simulink model "Comparison_with_prior_ESC_Methods"  (R2023a)
settings: Solver=ode4  StartTime=0.0  StopTime=500  FixedStep=0.0001  RelTol=1e-6
settings Model: Creator=Ahmed  LastModifiedBy=Ahmed

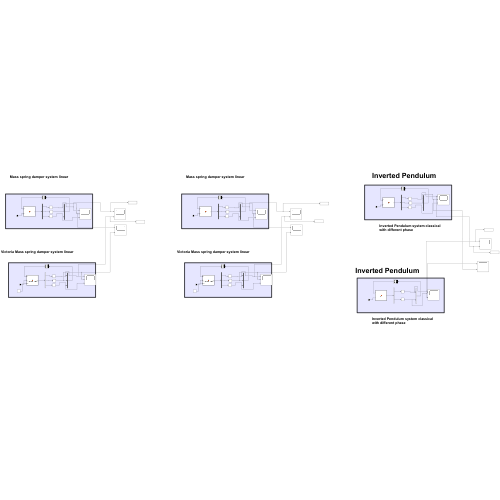
[thumbnail: Simulink's stored preview of the top-level diagram]
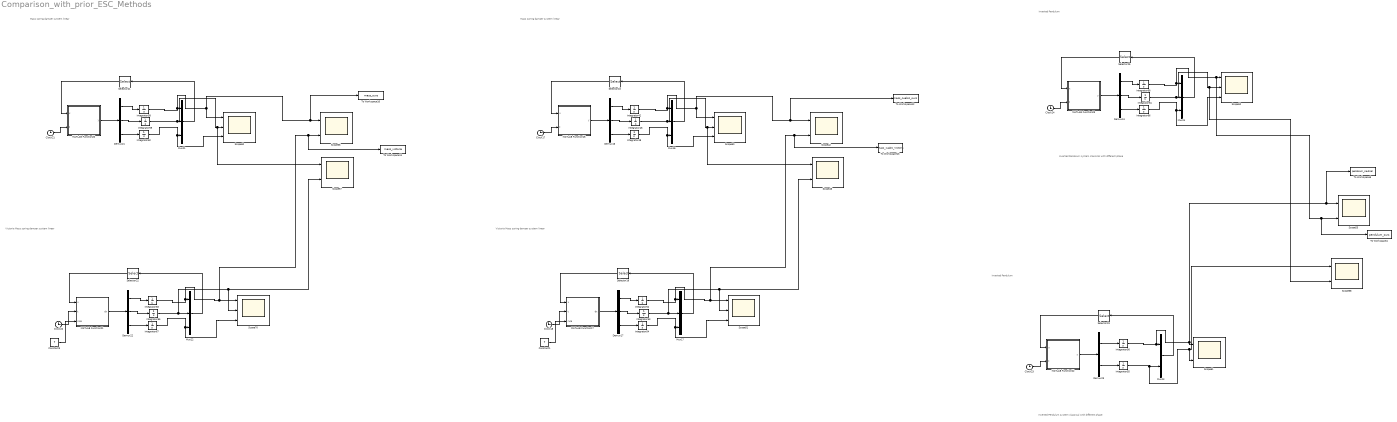
== system Comparison_with_prior_ESC_Methods ==
  note: Mass spring damper system linear
  note: Victoria Mass spring damper system linear
  note: Mass spring damper system linear
  note: Victoria Mass spring damper system linear
  note: Inverted Pendulum system classical with different phase
  note: Inverted Pendulum
  note: Inverted Pendulum system classical with different phase
  note: Inverted Pendulum
  Clock{17..18,21..24} (6 alike) : Clock
  Constant1 : Constant  Value=7
  Constant3 : Constant  Value=7
  Demux{16..17,21..22,24} (5 alike) : Demux  Outputs=3
  Demux23 : Demux  Outputs=2
  Integrator42 : Integrator  InitialCondition=2
  Integrator{46,53,55,59,61,65} (6 alike) : Integrator  InitialCondition=-1
  Integrator{48,54,62,66..67} (5 alike) : Integrator
  Integrator52 : Integrator  InitialCondition=1.68
  Integrator56 : Integrator  InitialCondition=3
  Integrator58 : Integrator  InitialCondition=2
  Integrator63 : Integrator  InitialCondition=1.68
  Integrator68 : Integrator  InitialCondition=3
  MATLAB Function16 : MATLAB Function  TreatAsAtomicUnit=on
  MATLAB Function17 : MATLAB Function  TreatAsAtomicUnit=on
  MATLAB Function20 : MATLAB Function  TreatAsAtomicUnit=on
  MATLAB Function21 : MATLAB Function  TreatAsAtomicUnit=on
  MATLAB Function22 : MATLAB Function  TreatAsAtomicUnit=on
  MATLAB Function23 : MATLAB Function  TreatAsAtomicUnit=on
  Mux{16..17,21..22,24} (5 alike) : Mux  Inputs=3
  Mux23 : Mux  Inputs=2
  Scope{42,46,53,56..58,61} (7 alike) : Scope  NumInputPorts=2
  Scope{50..52,62,70} (5 alike) : Scope  NumInputPorts=3
  Selector{16,19,21..22,25} (5 alike) : Selector  InputPortWidth=3  IndexOptions=Index vector (dialog)  Indices=[1 2 3]  OutputSizes=1
  Selector23 : Selector  InputPortWidth=2  IndexOptions=Index vector (dialog)  Indices=[1 2]  OutputSizes=1
  To Workspace10 : ToWorkspace  VariableName=mass_ours  SaveFormat=Timeseries  SampleTime=-1
  To Workspace11 : ToWorkspace  VariableName=mass_victoria  SaveFormat=Timeseries  SampleTime=-1
  To Workspace12 : ToWorkspace  VariableName=mass_cuabic_ours  SaveFormat=Timeseries  SampleTime=-1
  To Workspace13 : ToWorkspace  VariableName=mass_cuabic_Victoria  SaveFormat=Timeseries  SampleTime=-1
  To Workspace4 : ToWorkspace  VariableName=pendulum_ours  SaveFormat=Timeseries  SampleTime=-1
  To Workspace5 : ToWorkspace  VariableName=pendulum_sautner  SaveFormat=Timeseries  SampleTime=-1
  wires:
  Constant3/1 -> MATLAB Function21/3(rule)
  Demux22/1 -> Integrator63/1
  MATLAB Function21/1(dx) -> Demux22/1
  Demux22/3 -> Integrator67/1
  Demux22/2 -> Integrator65/1
  Clock22/1 -> MATLAB Function21/2(t)
  Mux22/1 -> Selector22/1
  Integrator67/1 -> Scope70/3, Mux22/3
  Selector22/1 -> MATLAB Function21/1(x)
  Integrator63/1 -> Mux22/1, Scope70/1, To Workspace11/1, Scope56/2
  Integrator65/1 -> Scope70/2, Scope57/2, Mux22/2
  Integrator59/1 -> Scope57/1, Scope62/2, Mux21/2
  Selector21/1 -> MATLAB Function20/1(x)
  Integrator62/1 -> Mux21/3, Scope62/3
  Mux21/1 -> Selector21/1
  Clock21/1 -> MATLAB Function20/2(t)
  Demux21/2 -> Integrator59/1
  Demux21/3 -> Integrator62/1
  MATLAB Function20/1(y) -> Demux21/1
  Demux21/1 -> Integrator58/1
  Demux16/1 -> Integrator42/1
  MATLAB Function16/1(y) -> Demux16/1
  Demux16/3 -> Integrator48/1
  Demux16/2 -> Integrator46/1
  Clock17/1 -> MATLAB Function16/2(t)
  Mux16/1 -> Selector16/1
  Integrator48/1 -> Scope50/3, Mux16/3
  Selector16/1 -> MATLAB Function16/1(x)
  Integrator42/1 -> Mux16/1, Scope50/1, To Workspace12/1, Scope42/1
  Integrator46/1 -> Mux16/2, Scope50/2, Scope46/1
  Integrator53/1 -> Mux17/2, Scope46/2, Scope51/2
  Integrator52/1 -> To Workspace13/1, Scope42/2, Scope51/1, Mux17/1
  Selector19/1 -> MATLAB Function17/1(x)
  Integrator54/1 -> Mux17/3, Scope51/3
  Mux17/1 -> Selector19/1
  Clock18/1 -> MATLAB Function17/2(t)
  Demux17/2 -> Integrator53/1
  Demux17/3 -> Integrator54/1
  MATLAB Function17/1(dx) -> Demux17/1
  Demux17/1 -> Integrator52/1
  Constant1/1 -> MATLAB Function17/3(rule)
  Integrator68/1 -> Mux24/1, Scope52/1, To Workspace4/1, Scope53/2
  MATLAB Function23/1(y) -> Demux24/1
  Clock24/1 -> MATLAB Function23/2(t)
  Selector25/1 -> MATLAB Function23/1(x)
  Integrator61/1 -> Mux24/2, Scope52/2, Scope58/2
  Mux24/1 -> Selector25/1
  Integrator66/1 -> Mux24/3, Scope52/3
  Demux24/2 -> Integrator61/1
  Demux24/1 -> Integrator68/1
  Demux24/3 -> Integrator66/1
  Demux23/1 -> Integrator56/1
  Demux23/2 -> Integrator55/1
  Mux23/1 -> Selector23/1
  Integrator56/1 -> Scope61/1, To Workspace5/1, Scope53/1, Mux23/1
  Integrator55/1 -> Mux23/2, Scope61/2, Scope58/1
  Selector23/1 -> MATLAB Function22/1(x)
  Clock23/1 -> MATLAB Function22/2(t)
  MATLAB Function22/1(y) -> Demux23/1
  Integrator58/1 -> To Workspace10/1, Scope56/1, Scope62/1, Mux21/1

== matlab function Comparison_with_prior_ESC_Methods/MATLAB Function16 ==
  data: x input; y output; t input
function y = fcn(x,t)

% Parameters for mass-spring-damper system
m = 1; % Mass
alpha = 10; % Spring constant
beta = 5; % Damping coefficient

c1=6;
a1=1;
% Define the system of equations as a function
omega=3.2;
k=0.72;
J=(x(1)-1)^2;


y = [
    x(2); 
    (-(alpha/m) * x(1) - (beta/m) * x(2)^3 + c1 * x(3)+ a1*omega*cos(omega*t)); 
    (k*J*omega*cos(omega*t)) ;
];

== matlab function Comparison_with_prior_ESC_Methods/MATLAB Function17 ==
  data: x input; dx output; t input; rule input
function dx = esc_example1_dynamics(x, t, rule)
% ESC dynamics for Simulink
% Inputs:
%   x = [x1; x2; u]
%   t = time (from Clock)
%   rule = 7, 8, or 9 for g1/g2 selection

% Parameters
k = 10;
mu = 5;

l_star = 1;
gamma = 100;
eps =1/12.3;
eta = 25;

% Extract states
x1 = x(1);
x2 = x(2);
u = x(3);

% Objective
y = x1 - l_star;
J = y^2;

% Frequency
freq = 2 * pi / (eta * sqrt(eps)^2);

% g1, g2 based on rule
switch rule
    case 7
        g1 = sqrt(gamma) * J;
        g2 = sqrt(gamma);
    case 8
        g1 = sqrt(gamma) * sin(J);
        g2 = sqrt(gamma);
    case 9
        g1 = sqrt(gamma) * sqrt(J);
        g2 = sqrt(gamma);
    otherwise
        g1 = 0;
        g2 = 0;
end

% ESC update law
du = (2 * sqrt(pi)) / (eta * sqrt(eps)) * (g1 * cos(freq * t) + g2 * sin(freq * t));

% System dynamics
dx1 = x2;
dx2 = -k * x1 - mu * x2^3 - u;
dx3 = du;

dx = [dx1; dx2; dx3];
end

== matlab function Comparison_with_prior_ESC_Methods/MATLAB Function20 ==
  data: x input; y output; t input
function y = fcn(x,t)

% Parameters for mass-spring-damper system
m = 1; % Mass
alpha = 10; % Spring constant
beta = 5; % Damping coefficient

c1=6;
a1=1;
% Define the system of equations as a function
omega=3.2;
k=0.72;
J=(x(1)-1)^2;


y = [
    x(2); 
    (-(alpha/m) * x(1) - (beta/m) * x(2) + c1 * x(3)+ a1*omega*cos(omega*t)); 
    (k*J*omega*cos(omega*t)) ;
];

== matlab function Comparison_with_prior_ESC_Methods/MATLAB Function21 ==
  data: x input; dx output; t input; rule input
function dx = esc_example1_dynamics(x, t, rule)
% ESC dynamics for Simulink
% Inputs:
%   x = [x1; x2; u]
%   t = time (from Clock)
%   rule = 7, 8, or 9 for g1/g2 selection

% Parameters
k = 10;
mu = 5;

l_star = 1;
gamma = 100;
eps =1/12.3;
eta = 25;

% Extract states
x1 = x(1);
x2 = x(2);
u = x(3);

% Objective
y = x1 - l_star;
J = y^2;

% Frequency
freq = 2 * pi / (eta * sqrt(eps)^2);

% g1, g2 based on rule
switch rule
    case 7
        g1 = sqrt(gamma) * J;
        g2 = sqrt(gamma);
    case 8
        g1 = sqrt(gamma) * sin(J);
        g2 = sqrt(gamma);
    case 9
        g1 = sqrt(gamma) * sqrt(J);
        g2 = sqrt(gamma);
    otherwise
        g1 = 0;
        g2 = 0;
end

% ESC update law
du = (2 * sqrt(pi)) / (eta * sqrt(eps)) * (g1 * cos(freq * t) + g2 * sin(freq * t));

% System dynamics
dx1 = x2;
dx2 = -k * x1 - mu * x2 - u;
dx3 = du;

dx = [dx1; dx2; dx3];
end

== matlab function Comparison_with_prior_ESC_Methods/MATLAB Function22 ==
  data: x input; y output; t input
function y = fcn(x,t)

% Parameters for mass-spring-damper system
m = 1; % Mass of the pendulum bob (kg)
L = 1; % Length of the pendulum rod (m)
g = 9.81; % Gravitational acceleration (m/s^2)
beta = 10; % Damping coefficient (Ns/m)
% Define the system of equations as a function

x_des = 2;

mu =14;
lambda =14;


omega = 50;

% Extract states

% Objective function
J = (x(1) - x_des)^2;

%J = -4 * exp(-norm(x(1)-1)^2 / 4);

% Shaping function
a = sqrt(J + log(2 * cosh(J)));

% Control law (no filter)
u = mu * a^2 + lambda * omega * sqrt(2)*sin(omega * t) * a + mu * a^2 + lambda * omega * sqrt(2)*cos(omega * t) * a;

y = [
    x(2); % dx1/dt = x2 (velocity)
    (g/L) * sin(x(1)) - (beta/(m*L)) * x(2) + u; % dx2/dt = acceleration with damping, spring force, and control input
];

== matlab function Comparison_with_prior_ESC_Methods/MATLAB Function23 ==
  data: x input; y output; t input
function y = fcn(x,t)

% Parameters for mass-spring-damper system
m = 1; % Mass of the pendulum bob (kg)
L = 1; % Length of the pendulum rod (m)
g = 9.81; % Gravitational acceleration (m/s^2)
beta = 10; % Damping coefficient (Ns/m)
% Define the system of equations as a function

c1=7;
k=1;
a1=1;

omega=50;
J=(x(1)-2)^2;

%J = -4 * exp(-norm(x(1)-1)^2 / 4);

y = [
    x(2); % dx1/dt = x2 (velocity)
    (g/L) * sin(x(1)) - (beta/(m*L)) * x(2) + c1 * x(3)+ a1*omega*cos(omega*t); % dx2/dt = acceleration with damping, spring force, and control input
    k*J*omega*cos(omega*t)
];
